simulink model "band_controller_sim"  (R2020b)
settings: Solver=FixedStepAuto  StartTime=0.0  StopTime=stop_time  RelTol=1e-3
InitFcn:
  | band_controller_sim_init
StopFcn:
  | band_controller_sim_stop
values from neighbouring files (symbols this model uses):
  fs = 128 * audio_fs    (= 6144000)    [band_controller_sim_init.m]
settings Model: Creator=t96f346  LastModifiedBy=conno
settings SolverCC: AutoInsertRateTranBlk=on
settings DataIOCC: ReturnWorkspaceOutputs=off
settings DebuggingCC: AlgebraicLoopMsg=error
settings ModelReferenceCC: EnableParallelModelReferenceBuilds=on  ParallelModelReferenceMATLABWorkerInit=Copy Base Workspace

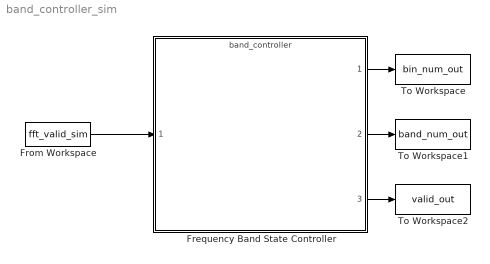
== system band_controller_sim ==
  Frequency Band State Controller : ModelReference  ModelNameDialog=band_controller.slx  SimulationMode=Normal  ModelReferenceVersion=2.45
  From Workspace : FromWorkspace  VariableName=fft_valid_sim  SampleTime=1/fs  Interpolate=off  OutputAfterFinalValue=Holding final value
  To Workspace : ToWorkspace  VariableName=bin_num_out  SampleTime=-1
      settings: Save2DSignal=2-D array (concatenate along first dimension)
  To Workspace1 : ToWorkspace  VariableName=band_num_out  SampleTime=-1
      settings: Save2DSignal=2-D array (concatenate along first dimension)
  To Workspace2 : ToWorkspace  VariableName=valid_out  SampleTime=-1
      settings: Save2DSignal=2-D array (concatenate along first dimension)
  wires:
  From Workspace/1 -> Frequency Band State Controller/1
  Frequency Band State Controller/3 -> To Workspace2/1
  Frequency Band State Controller/2 -> To Workspace1/1
  Frequency Band State Controller/1 -> To Workspace/1
